simulink model "sedemo_astable_multivibrator"  (Simulink 7.5)
settings: Solver=ode15s  StartTime=0.0  StopTime=2  RelTol=1e-3
model workspace (MAT data in the model file):
  Vcc = 6
  Gnd = 0
  R1 = 4700
  R2 = 4700
  C1 = 4.7e-06
  C2 = 4.7e-06
  turn_on_voltage = 0.6
  v_transient = -5.3999
InitFcn:
  | hws = get_param(bdroot, 'modelworkspace');
  | 
  | [R1 C1 R2 C2] = sedemo_init_multivibrator;
  | 
  | hws.assignin('R1', R1);
  | hws.assignin('C1', C1);
  | hws.assignin('R2', R2);
  | hws.assignin('C2', C2);
  | 
  | clear hws R1 C1 R2 C2
values from neighbouring files (symbols this model uses):
  C1 = 4.7*10^-6    (= 4.7e-06)    [sedemo_init_multivibrator.m]
  C2 = 4.7*10^-6    (= 4.7e-06)    [sedemo_init_multivibrator.m]
  R1 = 4.7*10^3    (= 4700)    [sedemo_init_multivibrator.m]
  R2 = 4.7*10^3    (= 4700)    [sedemo_init_multivibrator.m]
libraries: simeventssignalmanage1 x3, simeventssink1 x2, simeventsinfo x1
settings Model: Creator=The MathWorks Inc.  ExtModeAutoUpdateStatusClock=off
settings DataIOCC: SaveOutput=off  SignalLogging=off  SaveTime=off
settings OptimizationCC: InitFltsAndDblsToZero=on
settings DebuggingCC: SaveWithParameterizedLinksMsg=none  SignalResolutionControl=TryResolveAllWithWarning  SolverPrmCheckMsg=none  InheritedTsInSrcMsg=none  MultiTaskDSMMsg=warning  MultiTaskCondExecSysMsg=none  StrictBusMsg=Warning
settings RTWCC: IncludeERTFirstTime=on
settings GRTTargetCC: TargetFcnLib=ansi_tfl_tmw.mat
settings SimEventsCC: propDiagAttribOutput=1  propDiagFcnCallOutput=1  propDiagStatOutput=0

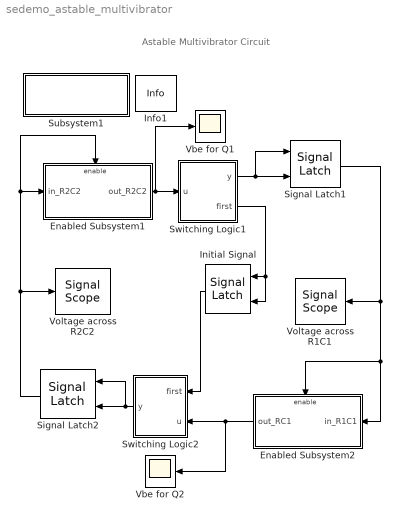
== system sedemo_astable_multivibrator ==
  note: Astable Multivibrator Circuit
  Enabled Subsystem1 : Subsystem  TreatAsAtomicUnit=on
      settings: PropExecContextOutsideSubsystem=on
  Enabled Subsystem2 : Subsystem  TreatAsAtomicUnit=on
      settings: PropExecContextOutsideSubsystem=on
  Info1 : simeventsinfo/Info  SystemSampleTime=-1
  Initial Signal : simeventssignalmanage1/Signal Latch  Priority=1  SystemSampleTime=-1  InitialMemoryValue=0  WriteMemoryUpon=Change in signal from port wvc  MemoryWriteEdgeOption=Either  SpecifyWriteEventPriority=on  PriorityMemoryWrite=1  ReadMemoryUpon=Write to memory event  MemoryReadEdgeOption=Falling  SpecifyReadEventPriority=on  PriorityMemoryRead=7000  ReportMemoryState=off  ReportMemoryUponWrite=on  ReportMemoryUponRead=off
  Signal Latch1 : simeventssignalmanage1/Signal Latch  Priority=1  SystemSampleTime=-1  InitialMemoryValue=Gnd  WriteMemoryUpon=Change in signal from port wvc  MemoryWriteEdgeOption=Either  SpecifyWriteEventPriority=on  PriorityMemoryWrite=350  ReadMemoryUpon=Write to memory event  MemoryReadEdgeOption=Falling  SpecifyReadEventPriority=on  PriorityMemoryRead=7000  ReportMemoryState=off  ReportMemoryUponWrite=on  ReportMemoryUponRead=off
  Signal Latch2 : simeventssignalmanage1/Signal Latch  Priority=1  SystemSampleTime=-1  InitialMemoryValue=Vcc  WriteMemoryUpon=Change in signal from port wvc  MemoryWriteEdgeOption=Either  SpecifyWriteEventPriority=on  PriorityMemoryWrite=7101  ReadMemoryUpon=Write to memory event  MemoryReadEdgeOption=Falling  SpecifyReadEventPriority=on  PriorityMemoryRead=7000  ReportMemoryState=off  ReportMemoryUponWrite=on  ReportMemoryUponRead=off
  Subsystem1 : Subsystem
      settings: OpenFcn=edit sedemo_init_multivibrator.m
      mask Display: disp('Change R,C values');
  Switching Logic1 : Subsystem  TreatAsAtomicUnit=on
  Switching Logic2 : Subsystem  TreatAsAtomicUnit=on
  Vbe for Q1 : Scope
      settings: TimeRange=2  YMin=-6  YMax=1
  Vbe for Q2 : Scope
      settings: TimeRange=2  YMin=-6  YMax=1
  Voltage across R1C1 : simeventssink1/Signal Scope  Priority=1  SystemSampleTime=-1  PlotType=Stair  InputType=Signal  NumInputs=1  AttributeNameY=Count  XInputOptionSignal=Event time  XInputOptionEntity=Event time  AttributeNameX=Count  EnableEntityOutport=on  XMin=0  XMax=1.84722438430489  XLimitExceededOption=Stretch axis limits  YLimitExceededOption=Stretch axis limits  AxisGrid=on  AxisLegend=off  LineDisables=""  LineColors=b  LineStyles=-  LineMarkers=*  OpenScopeAtSimStart=on  Title=Voltage across R1C1  YLabel=Voltage (V)  XLabel=Time (s)  FigurePosition=[760 218 229 198]  AxisZoom=off  DataStoreOption=Limited  DataPointsLimit=10000  StatNumberArrived=Off  ShowCountPlotted=off  ShowToolbar=off
      settings: YMin=0  YMax=6
  Voltage across R2C2 : simeventssink1/Signal Scope  Priority=1  SystemSampleTime=-1  PlotType=Stair  InputType=Signal  NumInputs=1  AttributeNameY=Count  XInputOptionSignal=Event time  XInputOptionEntity=Event time  AttributeNameX=Count  EnableEntityOutport=on  XMin=0  XMax=1.88722438430489  XLimitExceededOption=Stretch axis limits  YLimitExceededOption=Stretch axis limits  AxisGrid=on  AxisLegend=off  LineDisables=""  LineColors=b  LineStyles=-  LineMarkers=*  OpenScopeAtSimStart=on  Title=Voltage across R2C2  YLabel=Voltage (V)  XLabel=Time (s)  FigurePosition=[765 467 228 197]  AxisZoom=off  DataStoreOption=Limited  DataPointsLimit=10000  StatNumberArrived=Off  ShowCountPlotted=off  ShowToolbar=off
      settings: YMin=0  YMax=6
  wires:
  Enabled Subsystem1/1(out_R2C2) -> Switching Logic1/1(u), Vbe for Q1/1
  Signal Latch1/1 -> Voltage across R1C1/1, Enabled Subsystem2/Enable, Enabled Subsystem2/1(in_R1C1)
  Switching Logic1/2(first) -> Initial Signal/1, Initial Signal/2
  Switching Logic2/1(y) -> Signal Latch2/2, Signal Latch2/1
  Enabled Subsystem2/1(out_RC1) -> Switching Logic2/2(u), Vbe for Q2/1
  Initial Signal/1 -> Switching Logic2/1(first)
  Signal Latch2/1 -> Enabled Subsystem1/Enable, Enabled Subsystem1/1(in_R2C2), Voltage across R2C2/1
  Switching Logic1/1(y) -> Signal Latch1/2, Signal Latch1/1

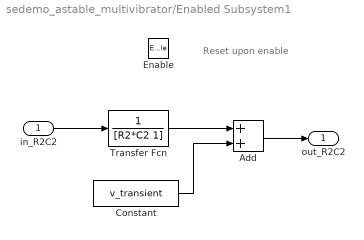
== system sedemo_astable_multivibrator/Enabled Subsystem1 ==
  note: Reset upon enable
  in_R2C2 : Inport  OutDataType=sfix(16)  OutScaling=2^0
  Enable : EnablePort  StatesWhenEnabling=reset
  Add : Sum  OutDataType=sfix(16)  OutScaling=2^-10
  Constant : Constant  Value=v_transient  OutDataType=sfix(16)  OutScaling=2^0  SampleTime=-1
  Transfer Fcn : TransferFcn  Denominator=[R2*C2 1]
  out_R2C2 : Outport  OutDataType=sfix(16)  OutScaling=2^0
  wires:
  in_R2C2/1 -> Transfer Fcn/1
  Transfer Fcn/1 -> Add/1
  Constant/1 -> Add/2
  Add/1 -> out_R2C2/1

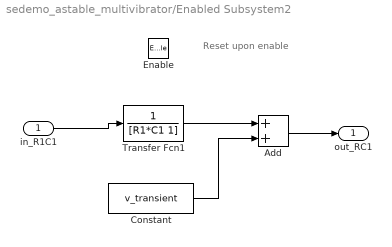
== system sedemo_astable_multivibrator/Enabled Subsystem2 ==
  note: Reset upon enable
  in_R1C1 : Inport  OutDataType=sfix(16)  OutScaling=2^0
  Enable : EnablePort  StatesWhenEnabling=reset
  Add : Sum  OutDataType=sfix(16)  OutScaling=2^-10
  Constant : Constant  Value=v_transient  OutDataType=sfix(16)  OutScaling=2^0  SampleTime=-1
  Transfer Fcn1 : TransferFcn  Denominator=[R1*C1 1]
  out_RC1 : Outport  OutDataType=sfix(16)  OutScaling=2^0
  wires:
  in_R1C1/1 -> Transfer Fcn1/1
  Constant/1 -> Add/2
  Transfer Fcn1/1 -> Add/1
  Add/1 -> out_RC1/1

== system sedemo_astable_multivibrator/Subsystem1 ==

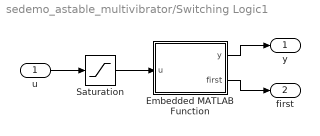
== system sedemo_astable_multivibrator/Switching Logic1 ==
  u : Inport  OutDataType=sfix(16)  OutScaling=2^0
  Embedded MATLAB Function : Stateflow chart  TreatAsAtomicUnit=on
  Saturation : Saturate  UpperLimit=turn_on_voltage  LowerLimit=v_transient
  y : Outport  OutDataType=sfix(16)  OutScaling=2^0
  first : Outport  Port=2  OutDataType=sfix(16)  OutScaling=2^0
  wires:
  u/1 -> Saturation/1
  Saturation/1 -> Embedded MATLAB Function/1(u)
  Embedded MATLAB Function/1(y) -> y/1
  Embedded MATLAB Function/2(first) -> first/1

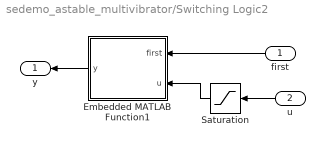
== system sedemo_astable_multivibrator/Switching Logic2 ==
  first : Inport  OutDataType=sfix(16)  OutScaling=2^0
  u : Inport  Port=2  OutDataType=sfix(16)  OutScaling=2^0
  Embedded MATLAB Function1 : Stateflow chart  TreatAsAtomicUnit=on
  Saturation : Saturate  UpperLimit=turn_on_voltage  LowerLimit=v_transient
  y : Outport  OutDataType=sfix(16)  OutScaling=2^0
  wires:
  first/1 -> Embedded MATLAB Function1/1(first)
  Embedded MATLAB Function1/1(y) -> y/1
  Saturation/1 -> Embedded MATLAB Function1/2(u)
  u/1 -> Saturation/1

== matlab function Switching Logic2/Embedded MATLAB Function1 ==
  settings: fimath=|
      | fimath(...
      | 'RoundMode', 'floor',...
      | 'OverflowMode', 'wrap',...
      | 'ProductMode', 'KeepLSB', 'ProductWordLength', 32,...
      | 'SumMode', 'KeepLSB', 'SumWordLength', 32,...
      | 'CastBeforeSum', false)
  data: first input double; u input double; y output double; Vcc parameter double; Gnd parameter double; turn_on_voltage parameter double
function y   = fcn(first, u, Vcc, Gnd, turn_on_voltage)
% This block supports an embeddable 
% subset of the MATLAB language.
% See the help menu for details.
if(first==0)
    y = Vcc;
else
    if(u>=turn_on_voltage)
       %If C1 is charged above the 
       % turn-on voltage, turn on Q2         
       y = Vcc;
    else
        y = Gnd;
    end
end

== matlab function Switching Logic1/Embedded MATLAB Function ==
  settings: fimath=|
      | fimath(...
      | 'RoundMode', 'floor',...
      | 'OverflowMode', 'wrap',...
      | 'ProductMode', 'KeepLSB', 'ProductWordLength', 32,...
      | 'SumMode', 'KeepLSB', 'SumWordLength', 32,...
      | 'CastBeforeSum', false)
  data: u input double; y output double; first output double; Vcc parameter double; Gnd parameter double; turn_on_voltage parameter double
function [y,first]  = fcn(u, Vcc, Gnd, turn_on_voltage)
% This block supports an embeddable 
% subset of the MATLAB language.
% See the help menu for details. 
persistent firstCall
if(isempty(firstCall))
   firstCall = 0;
end

if(u>=turn_on_voltage)
    % Processing that enables 
    % the Initial signal
    if(firstCall == 0)
        firstCall = 1;
    end
    first = 1;

    % If C2 is charged above the 
    % turn-on voltage, turn on Q1
    y = Vcc;
else
    first = 0;    
    y = Gnd;
end
